simulink subsystem "exp_ctrl_data_format"  (R2024a)
settings: Solver=VariableStepAuto  StartTime=0.0  StopTime=10.0  RelTol=1e-3
settings Model: Creator=gurt1  LastModifiedBy=gurt1

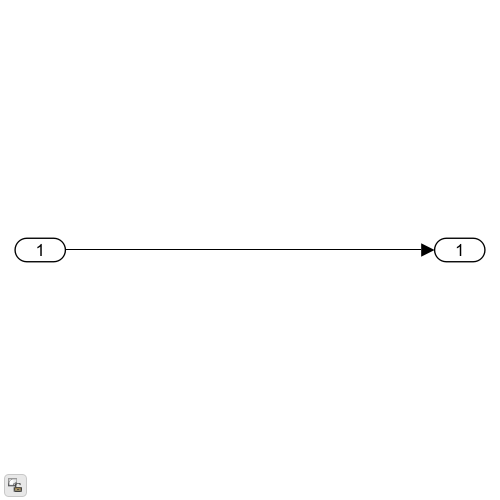
[thumbnail: Simulink's stored preview of the top-level diagram]
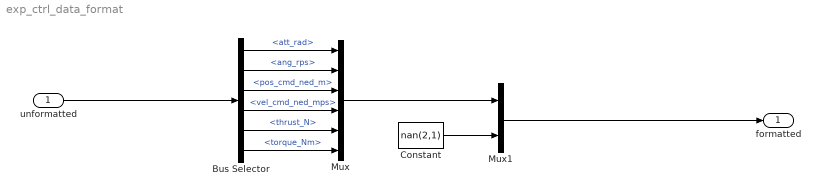
== system exp_ctrl_data_format ==
  unformatted : Inport
  Bus Selector : BusSelector  OutputSignals=exp_ctrl_data.OL_cmds.att_rad,exp_ctrl_data.OL_cmds.ang_rps,exp_ctrl_data.OL_data.pos_cmd_ned_m,exp_ctrl_data.OL_data.vel_cmd_ned_mps,exp_ctrl_data.OL_cmds.thrust_N,exp_ctrl_data.IL_cmds.torque_Nm
  Constant : Constant  Value=nan(2,1)
  Mux : Mux  Inputs=6
  Mux1 : Mux  Inputs=2
  formatted : Outport
  wires:
  unformatted/1 -> Bus Selector/1
  Bus Selector/1 -> Mux/1  "<att_rad>"
  Bus Selector/2 -> Mux/2  "<ang_rps>"
  Bus Selector/3 -> Mux/3  "<pos_cmd_ned_m>"
  Bus Selector/4 -> Mux/4  "<vel_cmd_ned_mps>"
  Bus Selector/5 -> Mux/5  "<thrust_N>"
  Bus Selector/6 -> Mux/6  "<torque_Nm>"
  Mux/1 -> Mux1/1
  Constant/1 -> Mux1/2
  Mux1/1 -> formatted/1
